simulink model "Ex2_1"  (R2019b)
settings: Solver=VariableStepAuto  StartTime=0.0  StopTime=10.0  RelTol=1e-3
values from neighbouring files (symbols this model uses):
  AAA = [ 0 0 0 1 0 0 0 0 0 0 0 0 ... (first row only)    [Ex2_1_constants.m]
  b = 0.001    [Ex2_1_constants.m]
  BBB = [0 0 0 0; 0 0 0 0; 0 0 0 0; 0 0 0 0; 0 0 0 0; help help help help; 0 0 0 0; 0 0 0 0; 0 0 0 0 ... (first row only)    [Ex2_1_constants.m]
  CCC = [ 1 0 0 0 0 0 0 0 0 0 0 0 ... (first row only)    [Ex2_1_constants.m]
  D = diag([kD, kD, kD])    [Ex2_1_constants.m]
  DDD = [0 0 0 0; 0 0 0 0; 0 0 0 0; 0 0 0 0; 0 0 0 0; 0 0 0 0]    [Ex2_1_constants.m]
  g_vec = [0, 0, -m*g]'    [Ex2_1_constants.m]
  I = diag([Ixx, Iyy, Izz])    [Ex2_1_constants.m]
  k = 0.01    [Ex2_1_constants.m]
  L = 0.225    [Ex2_1_constants.m]
  m = 0.5    [Ex2_1_constants.m]
  Omega = [0, 0, 0, 0]'    [Ex2_1_constants.m]
  omega_e = [tmp, tmp, tmp, tmp]'    [Ex2_1_constants.m]
libraries: vrlib x1
settings Model: Creator=ubuntu  LastModifiedBy=ubuntu

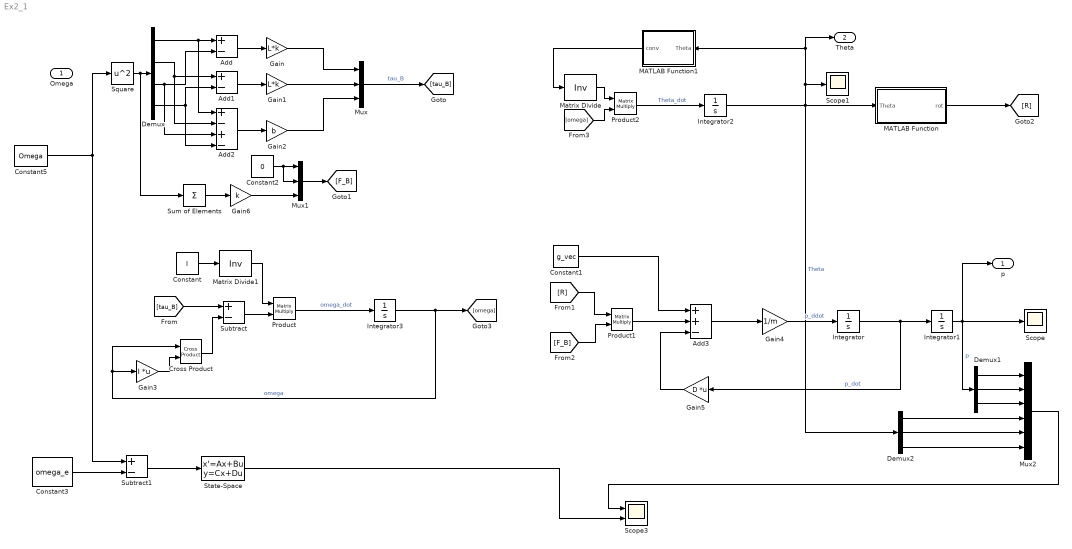
== system Ex2_1 ==
  Omega : Inport
  Add : Sum  Inputs=+-
  Add1 : Sum  Inputs=+-
  Add2 : Sum  Inputs=+-+-
  Add3 : Sum  Inputs=++-
  Constant : Constant  Value=I
  Constant1 : Constant  Value=g_vec
  Constant2 : Constant  Value=0
  Constant3 : Constant  Value=omega_e
  Constant5 : Constant  Value=Omega
  Cross Product : vrlib/Utilities/Cross Product
      settings: SourceProductName=Simulink
  Demux : Demux
  Demux1 : Demux  Outputs=3
  Demux2 : Demux  Outputs=3
  Gain : Gain  Gain=L*k
  Gain1 : Gain  Gain=L*k
  Gain2 : Gain  Gain=b
  Gain3 : Gain  Gain=I  Multiplication=Matrix(K*u)
  Gain4 : Gain  Gain=1/m
  Gain5 : Gain  Gain=D  Multiplication=Matrix(K*u)
  Gain6 : Gain  Gain=k
  Integrator : Integrator  InitialCondition=[0, 0, 0]'  ContinuousStateAttributes='p_dot'
  Integrator1 : Integrator  InitialCondition=[0, 0, 0]'  ContinuousStateAttributes='p'
  Integrator2 : Integrator  InitialCondition=[0, 0, 0]'  ContinuousStateAttributes='orientation'
  Integrator3 : Integrator  InitialCondition=[0, 0, 0]'  ContinuousStateAttributes='omega'
  MATLAB Function : MATLAB Function  TreatAsAtomicUnit=on
  MATLAB Function1 : MATLAB Function  TreatAsAtomicUnit=on
  Matrix Divide : Product  Inputs=/  Multiplication=Matrix(*)
  Matrix Divide1 : Product  Inputs=/  Multiplication=Matrix(*)
  Mux : Mux  Inputs=3
  Mux1 : Mux  Inputs=3
  Mux2 : Mux  Inputs=6
  Product : Product  Multiplication=Matrix(*)
  Product1 : Product  Multiplication=Matrix(*)
  Product2 : Product  Multiplication=Matrix(*)
  Scope : Scope
  Scope1 : Scope
  Scope3 : Scope  NumInputPorts=2
  Square : Math  Operator=square  SignedPower=off  SaturateOnIntegerOverflow=on
  State-Space : StateSpace  A=AAA  B=BBB  C=CCC  D=DDD  InitialCondition=[0,0,0,0,0,0,0,0,0,0,0,0]
  Subtract : Sum  Inputs=+-
  Subtract1 : Sum  Inputs=+-
  Sum of Elements : Sum  Inputs=+
  p : Outport
  "Theta " : Outport  Port=2
  wires:
  Gain4/1 -> Integrator/1  "p_ddot"
  Integrator/1 -> Gain5/1, Integrator1/1  "p_dot"
  Integrator1/1 -> Demux1/1, p/1, Scope/1  "p"
  Product2/1 -> Integrator2/1  "Theta_dot"
  Integrator2/1 -> Demux2/1, "Theta "/1, MATLAB Function1/1(Theta), Scope1/1, MATLAB Function/1(Theta)  "Theta"
  Product/1 -> Integrator3/1  "omega_dot"
  Add/1 -> Gain/1
  Demux/1 -> Add2/1, Add/1
  Demux/3 -> Add2/3, Add/2
  Add1/1 -> Gain1/1
  Demux/2 -> Add2/2, Add1/1
  Demux/4 -> Add1/2, Add2/4
  Add2/1 -> Gain2/1
  Gain1/1 -> Mux/2
  Gain/1 -> Mux/1
  Gain2/1 -> Mux/3
  Mux/1 -> [tau_B]  "tau_B"
  Subtract/1 -> Product/2
  [tau_B] -> Subtract/1
  Cross Product/1 -> Subtract/2
  Integrator3/1 -> [omega], Gain3/1, Cross Product/1  "omega"
  Gain3/1 -> Cross Product/2
  Gain5/1 -> Add3/3
  Sum of Elements/1 -> Gain6/1
  Gain6/1 -> Mux1/3
  Constant2/1 -> Mux1/1, Mux1/2
  Mux1/1 -> [F_B]
  Product1/1 -> Add3/2
  [R] -> Product1/1
  [F_B] -> Product1/2
  Matrix Divide/1 -> Product2/1
  [omega] -> Product2/2
  MATLAB Function1/1(conv) -> Matrix Divide/1
  Constant/1 -> Matrix Divide1/1
  Matrix Divide1/1 -> Product/1
  MATLAB Function/1(rot) -> [R]
  Square/1 -> Sum of Elements/1, Demux/1
  Constant1/1 -> Add3/1
  Add3/1 -> Gain4/1
  Mux2/1 -> Scope3/1
  State-Space/1 -> Scope3/2
  Demux2/3 -> Mux2/6
  Demux2/2 -> Mux2/5
  Demux2/1 -> Mux2/4
  Demux1/1 -> Mux2/1
  Demux1/2 -> Mux2/2
  Demux1/3 -> Mux2/3
  Subtract1/1 -> State-Space/1
  Constant3/1 -> Subtract1/2
  Constant5/1 -> Square/1, Subtract1/1

== matlab function Ex2_1/MATLAB Function1 ==
  data: Theta input; conv output
function conv = ConvMtx(Theta)

the = Theta(2);
phi = Theta(1);

conv = [1, 0, -sin(the); 0, cos(phi), cos(the)*sin(phi); 0, -sin(phi), cos(the)*cos(phi)];

== matlab function Ex2_1/MATLAB Function ==
  data: Theta input; rot output
function rot = RotMtx(Theta)

phi = Theta(1);
the = Theta(2);
psi = Theta(3);

rot = [
    cos(psi)*cos(the), cos(psi)*sin(the)*sin(phi)-sin(psi)*cos(phi), cos(psi)*sin(the)*cos(phi)+sin(psi)*sin(phi);
    sin(psi)*cos(the), sin(psi)*sin(the)*sin(phi)+cos(psi)*cos(phi), sin(psi)*sin(the)*cos(phi)-cos(psi)*sin(phi);
    -sin(the), cos(the)*sin(phi), cos(the)*cos(phi)
    ]';
